simulink model "ODU_zad3"  (Simulink 6.3)
settings: Solver=ode45  StartTime=0.0  StopTime=3  RelTol=1e-3
settings Model: LastModifiedBy=Ms1

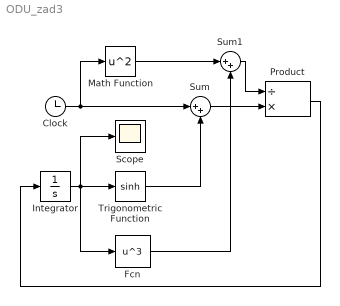
== system ODU_zad3 ==
  Clock : Clock
      settings: Decimation=10
  Fcn : Fcn  Expr=u^3
  Integrator : Integrator  InitialCondition=5
  Math Function : Math  Operator=square  SaturateOnIntegerOverflow=on
  Product : Product  Inputs=/*  SaturateOnIntegerOverflow=on  InputSameDT=on
  Scope : Scope
  Sum : Sum  Inputs=|++  SaturateOnIntegerOverflow=on  InputSameDT=on
  Sum1 : Sum  Inputs=|++  SaturateOnIntegerOverflow=on  InputSameDT=on
  Trigonometric Function : Trigonometry  Operator=sinh
  wires:
  Clock/1 -> Sum/1, Math Function/1
  Integrator/1 -> Trigonometric Function/1, Fcn/1, Scope/1
  Trigonometric Function/1 -> Sum/2
  Math Function/1 -> Sum1/1
  Fcn/1 -> Sum1/2
  Sum/1 -> Product/2
  Sum1/1 -> Product/1
  Product/1 -> Integrator/1
